simulink model "ljs20041"  (Simulink 2.20)
settings: Solver=ode45  StartTime=0.0  StopTime=50  RelTol=1e-3  AbsTol=1e-6
settings Model: ConsistencyChecking=off  RTWPlaceOutputsASAP=off

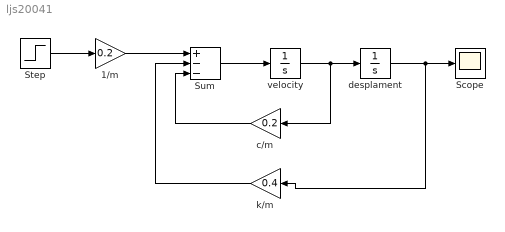
== system ljs20041 ==
  1/m : Gain  Gain=0.2
  Scope : Scope
      settings: TickLabels=on  TimeRange=auto  YMin=-5  YMax=5  SaveToWorkspace=off  SaveName=ScopeData
  Step : Step  Time=1  Before=0  After=1
  Sum : Sum  Inputs=+--
  c/m : Gain  Orientation=left  Gain=0.2
  desplament : Integrator  ExternalReset=none  InitialConditionSource=internal  InitialCondition=1  LimitOutput=off  UpperSaturationLimit=inf  LowerSaturationLimit=-inf  ShowSaturationPort=off  ShowStatePort=off  AbsoluteTolerance=auto
  k/m : Gain  Orientation=left  Gain=0.4
  velocity : Integrator  ExternalReset=none  InitialConditionSource=internal  InitialCondition=0  LimitOutput=off  UpperSaturationLimit=inf  LowerSaturationLimit=-inf  ShowSaturationPort=off  ShowStatePort=off  AbsoluteTolerance=auto
  wires:
  Sum/1 -> velocity/1
  velocity/1 -> desplament/1, c/m/1
  desplament/1 -> Scope/1, k/m/1
  1/m/1 -> Sum/1
  c/m/1 -> Sum/3
  k/m/1 -> Sum/2
  Step/1 -> 1/m/1
